simulink model "Neurofeedbac_Model_cute"  (R2022a)
settings: Solver=VariableStepAuto  StartTime=0.0  StopTime=75  RelTol=1e-3
libraries: fuzblock x1
settings Model: Creator=mariodelossantos  LastModifiedBy=mariodelossantos

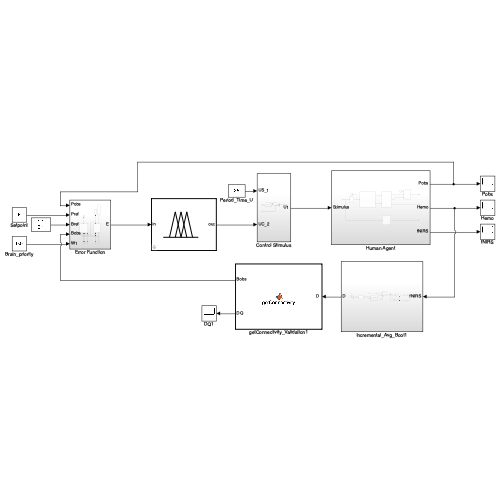
[thumbnail: Simulink's stored preview of the top-level diagram]
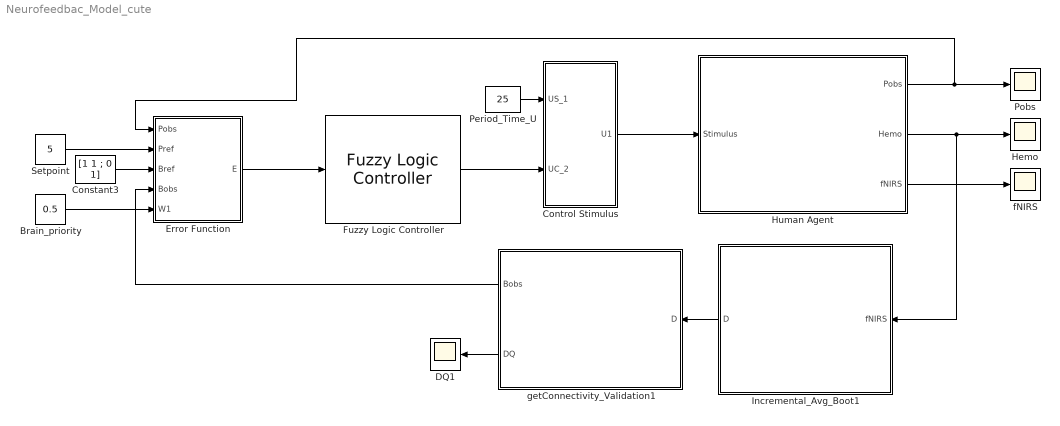
== system Neurofeedbac_Model_cute ==
  Brain_priority : Constant  Value=0.5
  Constant3 : Constant  Value="[1   1 ; 0  1]"
  Control Stimulus : Subsystem
  DQ1 : Scope
  Error Function : Subsystem
  Fuzzy Logic Controller : fuzblock/Fuzzy Logic  Controller  FIS=cFNIRS_c  OutputSampleNumber=101  DataType=double  FuzzifiedInputs=off  RuleFiringStrengths=off  RuleOutputs=off  AggregatedOutputs=off  SimulateUsing=Interpreted execution  OutOfRangeInputValueMessage=warning  NoRuleFiredMessage=warning  EmptyOutputFuzzySetMessage=warning
  Hemo : Scope
  Human Agent : Subsystem
  Incremental_Avg_Boot1 : Subsystem
  Period_Time_U : Constant  Value=25
  Pobs : Scope
  Setpoint : Constant  Value=5
  fNIRS : Scope
  getConnectivity_Validation1 : MATLAB Function  TreatAsAtomicUnit=on  SystemSampleTime=0
  wires:
  getConnectivity_Validation1/2(DQ) -> DQ1/1
  Incremental_Avg_Boot1/1("D ") -> getConnectivity_Validation1/1("D ")
  Period_Time_U/1 -> Control Stimulus/1(US_1)
  Error Function/1(E) -> Fuzzy Logic Controller/1
  Setpoint/1 -> Error Function/2(Pref)
  Fuzzy Logic Controller/1 -> Control Stimulus/2(UC_2)
  getConnectivity_Validation1/1(Bobs) -> Error Function/4(Bobs)
  Human Agent/3(fNIRS) -> fNIRS/1
  Human Agent/2(Hemo) -> Hemo/1, Incremental_Avg_Boot1/1(fNIRS)
  Human Agent/1(Pobs) -> Pobs/1, Error Function/1(Pobs)
  Control Stimulus/1(U1) -> Human Agent/1(Stimulus)
  Constant3/1 -> Error Function/3(Bref)
  Brain_priority/1 -> Error Function/5(W1)

== system Neurofeedbac_Model_cute/Control Stimulus ==
  US_1 : Inport
  UC_2 : Inport  Port=2
  Duty_Cycle_U1 : Constant  Value=0.26667  OutMin=[0]  OutMax=[0.8]
  Mux : Mux  Inputs=2
  Variable Pulse Generator2 : VariablePulseGenerator  RunAtFixedTimeIntervals=on  SampleTime=1/100
  U1 : Outport
  wires:
  Duty_Cycle_U1/1 -> Variable Pulse Generator2/1
  US_1/1 -> Variable Pulse Generator2/2
  Variable Pulse Generator2/1 -> Mux/1
  UC_2/1 -> Mux/2
  Mux/1 -> U1/1

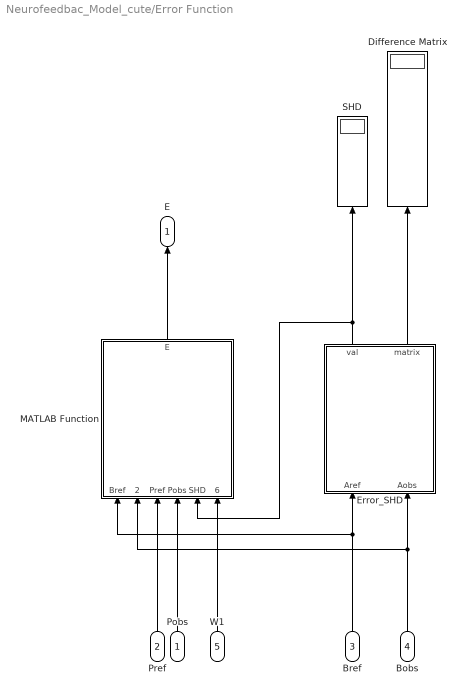
== system Neurofeedbac_Model_cute/Error Function ==
  Pobs : Inport
  Pref : Inport  Port=2
  Bref : Inport  Port=3
  Bobs : Inport  Port=4
  W1 : Inport  Port=5
  Difference Matrix : Display
  Error_SHD : MATLAB Function  TreatAsAtomicUnit=on
  MATLAB Function : MATLAB Function  TreatAsAtomicUnit=on
  SHD : Display
  E : Outport
  wires:
  Error_SHD/2(matrix) -> Difference Matrix/1
  Bref/1 -> Error_SHD/1(Aref), MATLAB Function/1(Bref)
  Error_SHD/1(val) -> MATLAB Function/5(SHD), SHD/1
  MATLAB Function/1(E) -> E/1
  Bobs/1 -> Error_SHD/2(Aobs), MATLAB Function/2(Bobs)
  Pobs/1 -> MATLAB Function/4(Pobs)
  Pref/1 -> MATLAB Function/3(Pref)
  W1/1 -> MATLAB Function/6(w1_input)

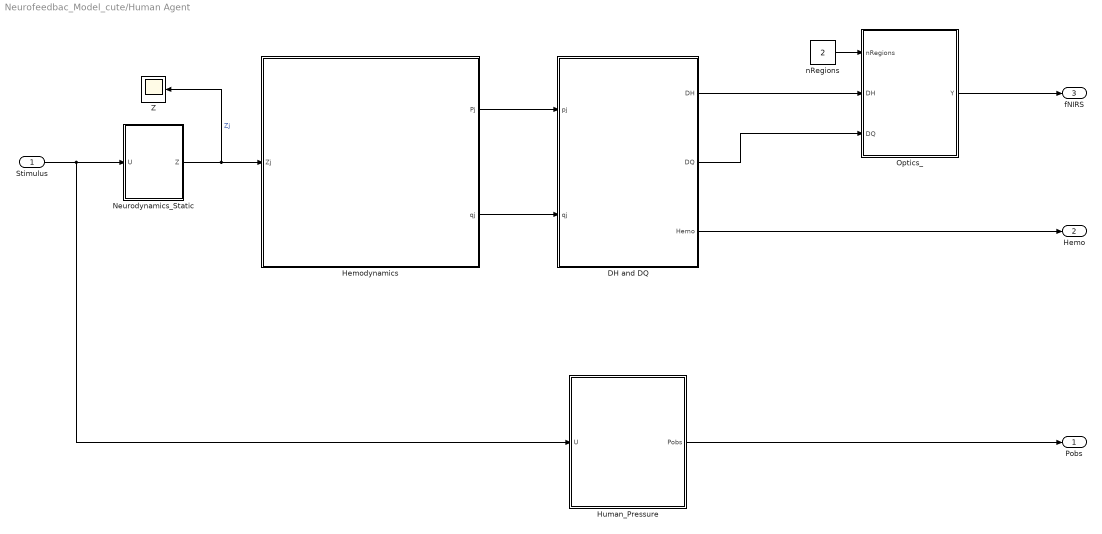
== system Neurofeedbac_Model_cute/Human Agent ==
  Stimulus : Inport
  DH and DQ : Subsystem
  Hemodynamics : Subsystem
  Human_Pressure : Subsystem
  Neurodynamics_Static : Subsystem
  Optics_ : MATLAB Function  TreatAsAtomicUnit=on
  Z : Scope
  nRegions : Constant  Value=2
  Pobs : Outport
  Hemo : Outport  Port=2
  fNIRS : Outport  Port=3
  wires:
  Hemodynamics/1(Pj) -> DH and DQ/1(pj)
  Hemodynamics/2(qj) -> DH and DQ/2(qj)
  DH and DQ/1(DH) -> Optics_/2(DH)
  DH and DQ/2(DQ) -> Optics_/3(DQ)
  Neurodynamics_Static/1(Z) -> Z/1, Hemodynamics/1(Zj)  "Zj"
  Stimulus/1 -> Human_Pressure/1(U), Neurodynamics_Static/1(U)
  nRegions/1 -> Optics_/1(nRegions)
  Optics_/1(Y) -> fNIRS/1
  DH and DQ/3(Hemo) -> Hemo/1
  Human_Pressure/1(Pobs) -> Pobs/1

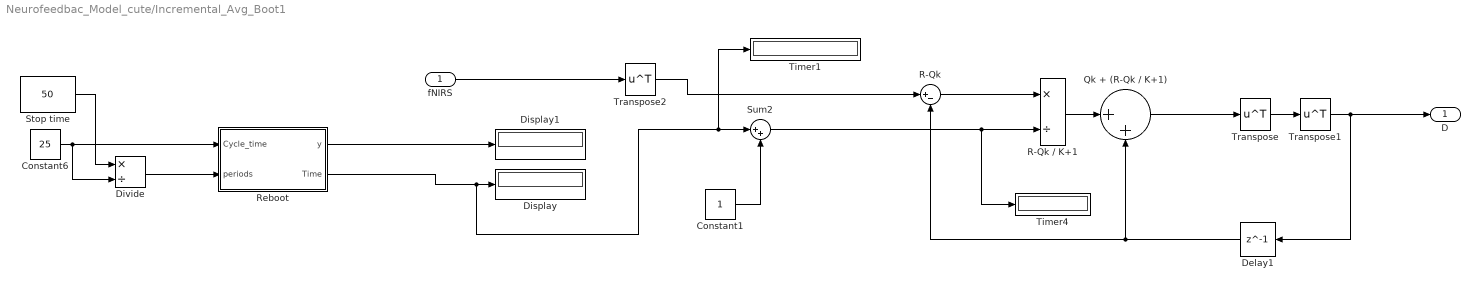
== system Neurofeedbac_Model_cute/Incremental_Avg_Boot1 ==
  fNIRS : Inport
  Constant1 : Constant
  Constant6 : Constant  Value=25
  Delay1 : Delay  DelayLength=1  InitialCondition=[0 0 0 0]
  Display : Display
  Display1 : Display
  Divide : Product  Inputs=*/
  "Qk + (R-Qk / K+1) " : Sum  Inputs=|++
  R-Qk : Sum  Inputs=|+-
  R-Qk / K+1 : Product  Inputs=*/
  Reboot : Subsystem
  Stop time : Constant  Value=50
  Sum2 : Sum  Inputs=|++
  Timer1 : Display
  Timer4 : Display
  Transpose : Math  Operator=transpose
  Transpose1 : Math  Operator=transpose
  Transpose2 : Math  Operator=transpose
  "D " : Outport
  wires:
  Constant1/1 -> Sum2/2
  Transpose2/1 -> R-Qk/1
  R-Qk / K+1/1 -> "Qk + (R-Qk / K+1) "/1
  fNIRS/1 -> Transpose2/1
  Sum2/1 -> Timer4/1, R-Qk / K+1/2
  R-Qk/1 -> R-Qk / K+1/1
  Delay1/1 -> R-Qk/2, "Qk + (R-Qk / K+1) "/2
  Reboot/2(Time) -> Timer1/1, Sum2/1, Display/1
  "Qk + (R-Qk / K+1) "/1 -> Transpose/1
  Constant6/1 -> Divide/2, Reboot/1(Cycle_time)
  Reboot/1(y) -> Display1/1
  Transpose/1 -> Transpose1/1
  Transpose1/1 -> Delay1/1, "D "/1
  Divide/1 -> Reboot/2(periods)
  Stop time/1 -> Divide/1

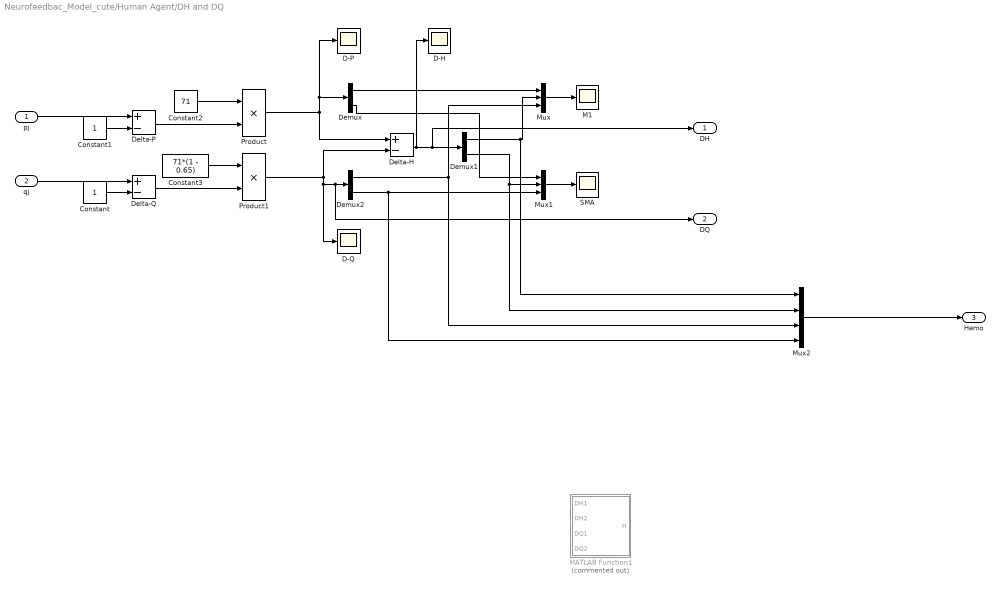
== system Neurofeedbac_Model_cute/Human Agent/DH and DQ ==
  pj : Inport
  qj : Inport  Port=2
  Constant : Constant
  Constant1 : Constant
  Constant2 : Constant  Value=71
  Constant3 : Constant  Value=71*(1 - 0.65)
  D-H : Scope
  D-P : Scope
  D-Q : Scope
  Delta-H : Sum  Inputs=+-
  Delta-P : Sum  Inputs=+-
  Delta-Q : Sum  Inputs=+-
  Demux : Demux  Outputs=2
  Demux1 : Demux  Outputs=2
  Demux2 : Demux  Outputs=2
  M1 : Scope
  MATLAB Function1 : MATLAB Function  Commented=on  TreatAsAtomicUnit=on
  Mux : Mux  Inputs=3
  Mux1 : Mux  Inputs=3
  Mux2 : Mux
  Product : Product
  Product1 : Product
  SMA : Scope
  DH : Outport
  DQ : Outport  Port=2
  Hemo : Outport  Port=3
  wires:
  Constant2/1 -> Product/1
  Delta-Q/1 -> Product1/2
  Constant3/1 -> Product1/1
  Demux2/2 -> Mux2/4, Mux1/3
  pj/1 -> Delta-P/1
  Mux1/1 -> SMA/1
  Demux/2 -> Mux1/1
  Mux/1 -> M1/1
  Constant/1 -> Delta-Q/2
  Delta-P/1 -> Product/2
  Product1/1 -> DQ/1, Demux2/1, D-Q/1, Delta-H/2
  qj/1 -> Delta-Q/1
  Demux/1 -> Mux/1
  Delta-H/1 -> DH/1, Demux1/1, D-H/1
  Demux1/1 -> Mux2/1, Mux/2
  Demux1/2 -> Mux2/2, Mux1/2
  Product/1 -> Demux/1, D-P/1, Delta-H/1
  Demux2/1 -> Mux2/3, Mux/3
  Constant1/1 -> Delta-P/2
  Mux2/1 -> Hemo/1

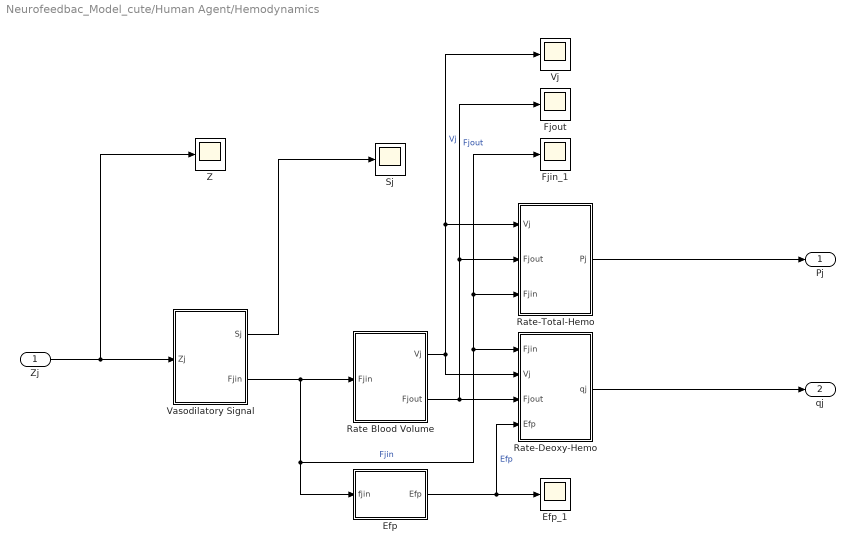
== system Neurofeedbac_Model_cute/Human Agent/Hemodynamics ==
  Zj : Inport
  Efp : MATLAB Function  TreatAsAtomicUnit=on
  Efp_1 : Scope
  Fjin_1 : Scope
  Fjout : Scope
  Rate Blood Volume : Subsystem
  Rate-Deoxy-Hemo : Subsystem
  Rate-Total-Hemo : Subsystem
  Sj : Scope
  Vasodilatory Signal : Subsystem
  Vj : Scope
  Z : Scope
  Pj : Outport
  qj : Outport  Port=2
  wires:
  Rate-Deoxy-Hemo/1(qj) -> qj/1
  Zj/1 -> Vasodilatory Signal/1(Zj), Z/1
  Vasodilatory Signal/1(Sj) -> Sj/1
  Rate Blood Volume/2(Fjout) -> Fjout/1, Rate-Total-Hemo/2(Fjout), Rate-Deoxy-Hemo/3(Fjout)  "Fjout"
  Rate Blood Volume/1(Vj) -> Vj/1, Rate-Total-Hemo/1(Vj), Rate-Deoxy-Hemo/2(Vj)  "Vj"
  Rate-Total-Hemo/1(Pj) -> Pj/1
  Efp/1(Efp) -> Rate-Deoxy-Hemo/4(Efp), Efp_1/1  "Efp"
  Vasodilatory Signal/2(Fjin) -> Efp/1(fjin), Fjin_1/1, Rate-Total-Hemo/3(Fjin), Rate-Deoxy-Hemo/1(Fjin), Rate Blood Volume/1(Fjin)  "Fjin"

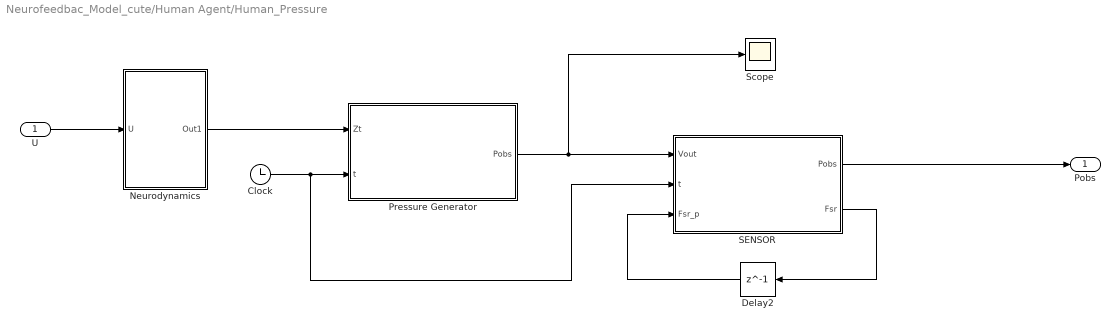
== system Neurofeedbac_Model_cute/Human Agent/Human_Pressure ==
  U : Inport
  Clock : Clock
  Delay2 : Delay  DelayLength=1  InitialCondition=0.0001
  Neurodynamics : Subsystem
  Pressure Generator : MATLAB Function  TreatAsAtomicUnit=on
  SENSOR : MATLAB Function  TreatAsAtomicUnit=on
  Scope : Scope
  Pobs : Outport
  wires:
  Clock/1 -> Pressure Generator/2(t), SENSOR/2(t)
  Delay2/1 -> SENSOR/3(Fsr_p)
  Pressure Generator/1(Pobs) -> Scope/1, SENSOR/1(Vout)
  SENSOR/2(Fsr) -> Delay2/1
  SENSOR/1(Pobs) -> Pobs/1
  U/1 -> Neurodynamics/1(U)
  Neurodynamics/1(Out1) -> Pressure Generator/1(Zt)

== system Neurofeedbac_Model_cute/Human Agent/Neurodynamics_Static ==
  U : Inport
  C : Gain  Gain=[0.08 0;0.06 0]  Multiplication=Matrix(K*u)
  Integrator : Integrator
  Jt : MATLAB Function  TreatAsAtomicUnit=on
  Sum : Sum  Inputs=|++
  Z : Outport
  wires:
  Integrator/1 -> Z/1, Jt/1(Zt)
  C/1 -> Sum/1
  Jt/1(Jt) -> Sum/2
  Sum/1 -> Integrator/1
  U/1 -> C/1, Jt/2(U)

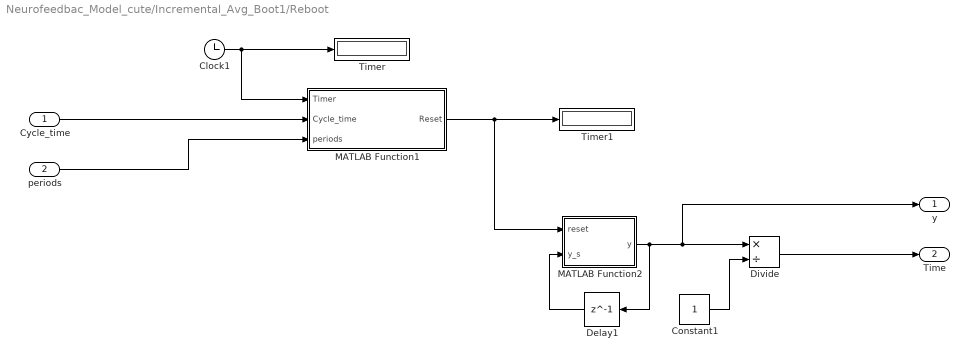
== system Neurofeedbac_Model_cute/Incremental_Avg_Boot1/Reboot ==
  Cycle_time : Inport
  periods : Inport  Port=2
  Clock1 : Clock
  Constant1 : Constant
  Delay1 : Delay  DelayLength=1
  Divide : Product  Inputs=*/
  MATLAB Function1 : MATLAB Function  TreatAsAtomicUnit=on
  MATLAB Function2 : MATLAB Function  TreatAsAtomicUnit=on
  Timer : Display
  Timer1 : Display
  y : Outport
  Time : Outport  Port=2
  wires:
  MATLAB Function1/1(Reset) -> MATLAB Function2/1(reset), Timer1/1
  MATLAB Function2/1(y) -> y/1, Divide/1, Delay1/1
  Constant1/1 -> Divide/2
  Clock1/1 -> MATLAB Function1/1(Timer), Timer/1
  periods/1 -> MATLAB Function1/3(periods)
  Delay1/1 -> MATLAB Function2/2(y_s)
  Divide/1 -> Time/1
  Cycle_time/1 -> MATLAB Function1/2(Cycle_time)

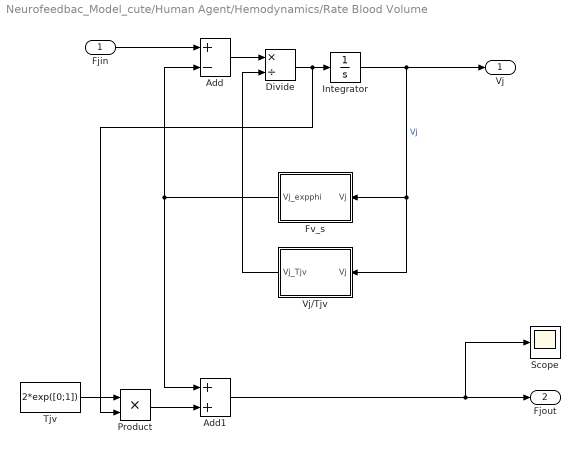
== system Neurofeedbac_Model_cute/Human Agent/Hemodynamics/Rate Blood Volume ==
  Fjin : Inport
  Add : Sum  Inputs=+-
  Add1 : Sum
  Divide : Product  Inputs=*/
  Fv_s : MATLAB Function  TreatAsAtomicUnit=on
  Integrator : Integrator  InitialCondition=exp([0;0])
  Product : Product
  Scope : Scope
  Tjv : Constant  Value=2*exp([0;1])
  Vj/Tjv : MATLAB Function  TreatAsAtomicUnit=on
  Vj : Outport
  Fjout : Outport  Port=2
  wires:
  Fjin/1 -> Add/1
  Integrator/1 -> Vj/1, Vj/Tjv/1(Vj), Fv_s/1(Vj)  "Vj"
  Divide/1 -> Product/2, Integrator/1
  Fv_s/1(Vj_expphi) -> Add/2, Add1/1
  Add/1 -> Divide/1
  Vj/Tjv/1(Vj_Tjv) -> Divide/2
  Product/1 -> Add1/2
  Tjv/1 -> Product/1
  Add1/1 -> Scope/1, Fjout/1

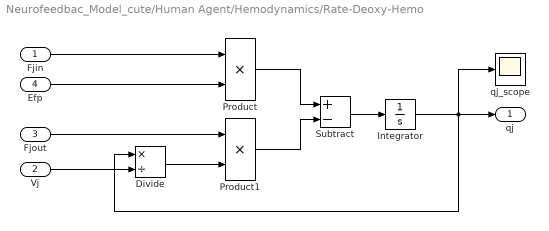
== system Neurofeedbac_Model_cute/Human Agent/Hemodynamics/Rate-Deoxy-Hemo ==
  Fjin : Inport
  Vj : Inport  Port=2
  Fjout : Inport  Port=3
  Efp : Inport  Port=4
  Divide : Product  Inputs=*/
  Integrator : Integrator  InitialCondition=exp([0;0])
  Product : Product
  Product1 : Product
  Subtract : Sum  Inputs=+-
  qj_scope : Scope
  qj : Outport
  wires:
  Efp/1 -> Product/2
  Divide/1 -> Product1/2
  Subtract/1 -> Integrator/1
  Integrator/1 -> qj/1, Divide/1, qj_scope/1
  Vj/1 -> Divide/2
  Product1/1 -> Subtract/2
  Fjin/1 -> Product/1
  Fjout/1 -> Product1/1
  Product/1 -> Subtract/1

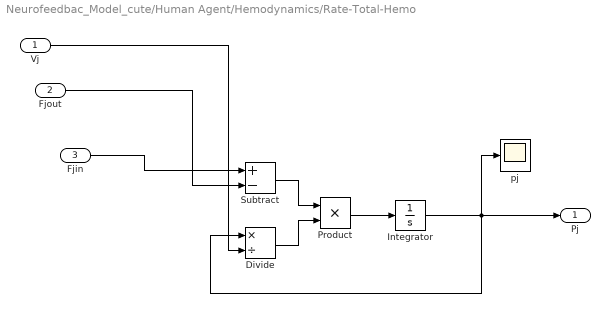
== system Neurofeedbac_Model_cute/Human Agent/Hemodynamics/Rate-Total-Hemo ==
  Vj : Inport
  Fjout : Inport  Port=2
  Fjin : Inport  Port=3
  Divide : Product  Inputs=*/
  Integrator : Integrator  InitialCondition=exp([0;0])
  Product : Product
  Subtract : Sum  Inputs=+-
  pj : Scope
  Pj : Outport
  wires:
  Fjout/1 -> Subtract/2
  Product/1 -> Integrator/1
  Vj/1 -> Divide/2
  Subtract/1 -> Product/1
  Fjin/1 -> Subtract/1
  Divide/1 -> Product/2
  Integrator/1 -> Pj/1, pj/1, Divide/1

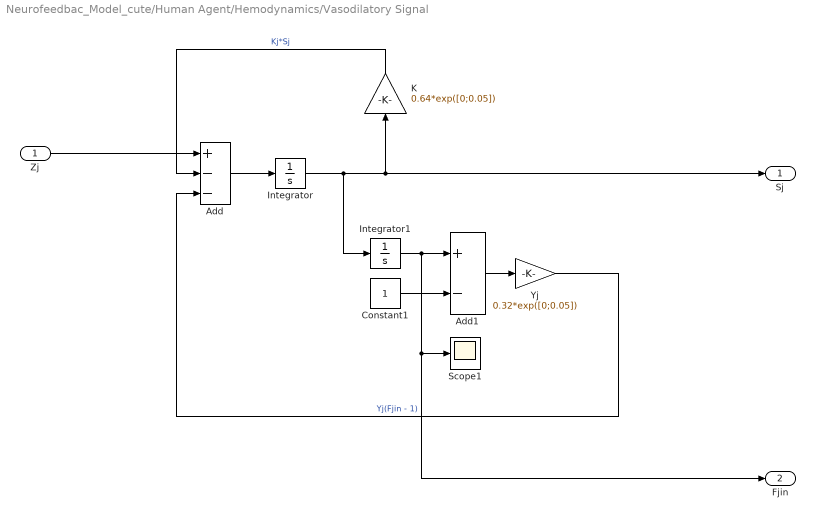
== system Neurofeedbac_Model_cute/Human Agent/Hemodynamics/Vasodilatory Signal ==
  Zj : Inport
  Add : Sum  Inputs=+--
  Add1 : Sum  Inputs=+-
  Constant1 : Constant
  Integrator : Integrator
  Integrator1 : Integrator  InitialCondition=exp([0;0])
  K : Gain  Gain=0.64*exp([0;0.05])
  Scope1 : Scope
  Yj : Gain  Gain=0.32*exp([0;0.05])
  Sj : Outport
  Fjin : Outport  Port=2
  wires:
  Add1/1 -> Yj/1
  K/1 -> Add/2  "Kj*Sj"
  Constant1/1 -> Add1/2
  Zj/1 -> Add/1
  Integrator1/1 -> Fjin/1, Scope1/1, Add1/1
  Integrator/1 -> Sj/1, K/1, Integrator1/1
  Add/1 -> Integrator/1
  Yj/1 -> Add/3  "Yj(Fjin - 1)"

== system Neurofeedbac_Model_cute/Human Agent/Human_Pressure/Neurodynamics ==
  U : Inport
  C1 : Gain  Gain=[0.08 0;0.06 0]  Multiplication=Matrix(K*u)
  Integrator1 : Integrator
  Jt1 : MATLAB Function  TreatAsAtomicUnit=on
  MATLAB Function : MATLAB Function  TreatAsAtomicUnit=on
  Sum1 : Sum  Inputs=|++
  Out1 : Outport
  wires:
  Jt1/1(Jt) -> Sum1/2
  C1/1 -> Sum1/1
  U/1 -> MATLAB Function/1(U)
  Integrator1/1 -> Out1/1, Jt1/1(Zt)
  MATLAB Function/1(Up) -> C1/1, Jt1/2(U)
  Sum1/1 -> Integrator1/1

== matlab function Neurofeedbac_Model_cute/Human Agent/Human_Pressure/SENSOR ==
  data: Vout input; Pobs output; t input; Fsr_p input; Fsr output
function [Pobs,Fsr] = PressureGenerator_sensor(Vout, t,Fsr_p)

    Vcc = 50; %Considering 5V as a real sensor, the value is on mV
    Rf = 100; %Fixed resistor 10k ohms
    kgf = 0.1019716213; % 1N = 0.1019716213 kgf
    Fsr = 0;
    Fsrforce = 0;
    Fsr = (Vcc - Vout * Rf) / Vout;
    FsConductance = 1000000; %Sensor conductance in uOhms
    FsConductance = FsConductance / Fsr;
    if FsConductance <= 1000
        Fsrforce = FsConductance / 80; %Force on Newtons
    else
        Fsrforce = FsConductance - 1000;
        Fsrforce = Fsrforce / 30;
    end
    
Pobs = Fsrforce * kgf;

end

== matlab function Neurofeedbac_Model_cute/Human Agent/DH and DQ/MATLAB Function1 ==
  data: DH1 input; H output; DH2 input; DQ1 input; DQ2 input
function H = hemo(DH1, DH2, DQ1, DQ2)
H = zeros(1,4);

H(1,1) = DQ1;
H(1,2) = DQ2;
H(1,3) = DH1;
H(1,4) = DH2;

== matlab function Neurofeedbac_Model_cute/Incremental_Avg_Boot1/Reboot/MATLAB Function1 ==
  data: Timer input; Reset output; Cycle_time input; periods input
function Reset  = fcn(Timer, Cycle_time, periods)

temp = 0;
PCycles = zeros(periods,1);
for i = 1:periods
    PCycles(i) = i * Cycle_time;
    if (Timer >= PCycles(i) && Timer <= PCycles(i)+1)
        temp = 1;
        break
    else
        temp = 0;
    end
end 
Reset = temp;

== matlab function Neurofeedbac_Model_cute/Human Agent/Human_Pressure/Neurodynamics/MATLAB Function ==
  data: U input; Up output
function Up = fcn(U)
Up = zeros(2,1);
Up(1) = U(1);
Up(2) = U(2)*10;

== matlab function Neurofeedbac_Model_cute/Human Agent/Hemodynamics/Efp ==
  data: fjin input; Efp output
function Efp= fcn(fjin)

Efp = (1 - (1 - 0.32).^ (1 ./ fjin))/0.32;

== matlab function Neurofeedbac_Model_cute/Human Agent/Hemodynamics/Rate Blood Volume/Fv_s ==
  data: Vj input; Vj_expphi output
function Vj_expphi = fcn(Vj)
phi = 0.32;
Vj_expphi = Vj.^(1/phi);

== matlab function Neurofeedbac_Model_cute/Error Function/Error_SHD ==
  data: Aref input; val output; Aobs input; matrix output
function [val,matrix]=SHD(Aref,Aobs)

val = sum(sum(xor(Aref,Aobs)));
matrix = xor(Aref,Aobs);

== matlab function Neurofeedbac_Model_cute/Human Agent/Hemodynamics/Rate Blood Volume/Vj//Tjv ==
  data: Vj input; Vj_Tjv output
function Vj_Tjv = fcn(Vj)
    Tjv = 2*exp([0;1]);
    Tj = 2*exp([0;0.05]);
Vj_Tjv =(Tj.*Tjv.*Vj);

== matlab function Neurofeedbac_Model_cute/Error Function/MATLAB Function ==
  data: Bref input; E output size=1; Bobs input; Pref input; Pobs input; SHD input; w1_input input
function E  = ErrorFunction(Bref, Bobs, Pref, Pobs, SHD, w1_input)

    E = 0;
    w1 = w1_input; %Use whatever values you like most. Threshold 

    w2 = 1 - w1;

    assert(all(size(Bref) == size(Bobs)));

    assert(size(Bref,1) == size(Bref,2));

    nChannels = size(Bref,1);

    BfullyConnected = ones(nChannels);

    BfullyDisconnected = zeros(nChannels);

    maxDiffSHD = sum(sum(xor(BfullyConnected,BfullyDisconnected))); %SHD

    errA = SHD/maxDiffSHD; %Normalize error in the connectivity

    errP = abs(Pref-Pobs)/Pref;

    
E = w1 * errA + w2 * errP;

== matlab function Neurofeedbac_Model_cute/getConnectivity_Validation1 ==
  data: D input; Bobs output; DQ output
function [Bobs,DQ]  = getConnectivity(D)

    DQ = zeros(1, 2);
    DQ(1,1)=D(1,1);
    DQ(1,2)=D(1,2);


    DH = zeros(1,2);
    DH(1,1)=D(1,3);
    DH(1,2)=D(1,4);

    rThresh= 0.6; % [0..1] A threshold on the correlation.

    [nSamples,nChannels, nHb]=size(DQ);

    C = nan(nChannels, nChannels, nHb); %Matrix of channel pairwise correlations;

    %This part of the algorithm is HIGHLY inefficient but it does the job for now
    %but might not be sufficiently fast for "real time" neurofeedback

    for iHb = 1:nHb
        for iCh=1:nChannels
            for jCh=iCh:nChannels

                if iCh == jCh

                 C(iCh,jCh,iHb) = 1;

                else

                 C(iCh,jCh,iHb) = xcorr2(DQ(:,iCh,iHb),DQ(:,jCh,iHb));

                end
            end

        end

    end

    %Threshold/Binarize C


    tmp = C > rThresh;

    %Finally "merge" accross Hb species

    Bobs = all(tmp,3); %Apply the AND function across Hb species.

== matlab function Neurofeedbac_Model_cute/Human Agent/Neurodynamics_Static/Jt ==
  data: Zt input; U input; Jt output
function Jt = fcn(Zt, U)
   A = [-0.16 -0.49;-0.02 -0.33];
   nRegions  = size(A,1);
   M = size(U,1); %nStimuli
   simulationLength = size(U,2);
   B = zeros(2,2,2);
   B1 = [0 0; 0 0]; %There must be a B per stimulus
   B2 = [-0.02 -0.77; 0.33 -1.31];
   %B2 = [1 1; 1 1];
   B(:,:,1) = B1;
   B(:,:,2) = B2;
      assert(M == size(B,3),...
       'Unexpected number of induced connectivity parameters B.');
   T = zeros(nRegions); %nRegions x nRegions
    for t = 1:simulationLength
           for uu = 1:M % Sum (Uj * Bj)
               tmp = U(uu,t)*B(:,:,uu);
               T = -0.5*exp(T + tmp);  
           end
    end
    SI = diag(A);
    A =  A - diag(exp(SI) + (SI));
Jt = (A*Zt) + (T*Zt);

== matlab function Neurofeedbac_Model_cute/Incremental_Avg_Boot1/Reboot/MATLAB Function2 ==
  data: reset input; y_s input; y output
function y = fcn(reset, y_s)

if reset == 1
    y = 0;
else 
    y = (y_s + 1);
end

== matlab function Neurofeedbac_Model_cute/Human Agent/Human_Pressure/Neurodynamics/Jt1 ==
  data: Zt input; U input; Jt output
function Jt = fcn(Zt, U)
   A = [-0.16 -0.49;-0.02 -0.33];
   nRegions  = size(A,1);
   M = size(U,1); %nStimuli
   simulationLength = size(U,2);
   B = zeros(2,2,2);
   B1 = [0 0; 0 0]; %There must be a B per stimulus
   B2 = [-0.02 -0.77; 
          0.33 -1.31];
   %B2 = [1 1; 1 1];
   B(:,:,1) = B1;
   B(:,:,2) = B2;
      assert(M == size(B,3),...
       'Unexpected number of induced connectivity parameters B.');
   T = zeros(nRegions); %nRegions x nRegions
    for t = 1:simulationLength
           for uu = 1:M % Sum (Uj * Bj)
               tmp = U(uu,t)*B(:,:,uu);
               T = -0.5*exp(T + tmp);  
           end
    end
    SI = diag(A);
    A =  A - diag(exp(SI) + (SI));
Jt = (A*Zt) + (T*Zt);

== matlab function Neurofeedbac_Model_cute/Human Agent/Optics_ ==
  data: nRegions input; DH input; DQ input; Y output
function Y = Optical_Changes(nRegions,DH, DQ)
%% Version V1
% Authors - Mario De Los Santos, Felipe Orihuela-Espina, Javier Herrara-Vega
% Date - March, 2022
% Email - madlsh3517@gmail.com
% Based on: 2015 Stak DCM for fNIRS.
%
%% Input Parameters
% DQ - HbR - Rate of deoxy-hemoglobin
% DH - HbT - Total Hemoglobin
%
%% Output Parameters
% y- optical density changes 
%
%% 

%Using simulink is not possible to have a dynamic matrix that we can
%iterate based on the nRegions variable, but you could easly replace the
%number of regions in the variable "Regions" according your needs
Regions = 2;
Y = zeros(Regions,Regions);
tempDHQ = zeros(nRegions, 2);


% We are using as L1 = 780nm and as L2 = 850nm (same as STak for the
% second one)
%Based on: Giannoni, L., Lange, F., & Tachtsidis, I. (2020). Investigation of the quantification 
% of hemoglobin and cytochrome-c-oxidase in the exposed cortex with near-infrared hyperspectral imaging: 
% a simulation study. Journal of biomedical optics, 25(4), 046001.

F_P =[(0.0007358251*7.5) (0.001104715*6.5) ; (0.001159306*7.5) (0.0007858993*6.5)]; 

%Itereation between regions, nRegions is given as constant by the user.
for i = 1:nRegions
    tempDHQ(:,i) = DQ(i);
    tempDHQ(:,i) = DH(i);
    Y(:,:) = F_P * tempDHQ;
end

== matlab function Neurofeedbac_Model_cute/Human Agent/Human_Pressure/Pressure Generator ==
  data: Zt input; Pobs output; t input
function Pobs = fcn(Zt, t)
    R=10000; %Resistor [Ohms];
    C= 2; %Capacitor [Faradays];
    V= Zt(1); %Voltage or system reference;
    Vc = V * (exp(-t/(R*C))); % Voltage at the capacitor  
    
Pobs = Vc;
